simulink model "bldc_model_bst"  (R2014b)
settings: Solver=ode4  StartTime=0.0  StopTime=5  FixedStep=0.01  RelTol=1e-3
undefined symbols (not defined in the file or in its folder): spd_0
libraries: simulink x2
settings Model: Creator=root  LastModifiedBy=root

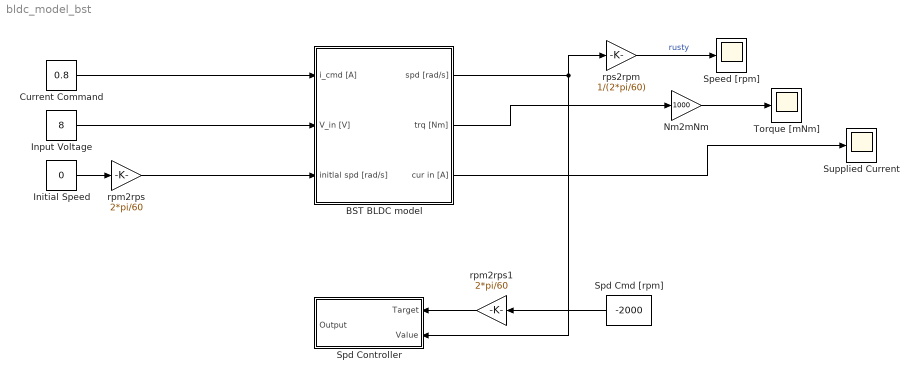
== system bldc_model_bst ==
  BST BLDC model : Subsystem  mask{Ke=1.026E-3/(2*pi/60), Km=1/96.154, R=2.3, frctn_c=[-3.77e-09, -1.42e-06, -6.76e-04], frctn_p=[-3.39e-09, -1.57e-06, -5.89e-04], frctn_n=[-9.44e-09, -4.31e-05, +3.57e-04], J=978.548e-6, i_max=0.9, V_in=8.0}
      mask prompts: Ke "Back-EMF Constant [V/(rad/s)]"; Km "Motor Torque Constant [Nm/A]"; R "Motor Resistance [Ohm]"; frctn_c "Friction Coefficients"; frctn_p "Friction Coefficients Pos"; frctn_n "Friction Coefficients Neg"; J "Moment of Inertia [kgm2]"; i_max "Maximum Current [A]"; V_in "Input Voltage [V]"
  "Current Command " : Constant  Value=0.8
  Initial Speed : Constant  Value=0
  Input Voltage : Constant  Value=8
  Nm2mNm : Gain  Gain=1000
  Spd Cmd [rpm] : Constant  Value=-2000
  Spd Controller : Subsystem  mask{kp=100E-3, ki=3.0e-05, kd=0.0, output_max=0.9}
      mask prompts: kp "Proportional Gain"; ki "Integrator Gain"; kd "Derivative Gain"; output_max "Maximum Output"
      mask DialogControl DescTextVar Prompt: This is a general PID controller with propotional gains, derivative gain and integral gain
  "Speed [rpm] " : Scope
      settings: ShowLegends=on  TimeRange=5  YMin=0  YMax=400
  Supplied Current : Scope
      settings: ShowLegends=on  TimeRange=10  YMin=0.344  YMax=0.351  SaveName=ScopeData2
  Torque [mNm] : Scope
      settings: ShowLegends=on  TimeRange=300  YMin=-20  YMax=20
  rpm2rps : Gain  Gain=2*pi/60
  rpm2rps1 : Gain  Gain=2*pi/60
  rps2rpm : Gain  Gain=1/(2*pi/60)
  wires:
  "Current Command "/1 -> BST BLDC model/1(i_cmd [A])
  BST BLDC model/1(spd [rad/s]) -> rps2rpm/1, Spd Controller/2(Value)
  rps2rpm/1 -> "Speed [rpm] "/1  "rusty"
  Input Voltage/1 -> BST BLDC model/2(V_in [V])
  Initial Speed/1 -> rpm2rps/1
  rpm2rps/1 -> BST BLDC model/3(initlal spd [rad/s])
  BST BLDC model/2(trq [Nm]) -> Nm2mNm/1
  Nm2mNm/1 -> Torque [mNm]/1
  BST BLDC model/3(cur in [A]) -> Supplied Current/1
  Spd Cmd [rpm]/1 -> rpm2rps1/1
  rpm2rps1/1 -> Spd Controller/1(Target)

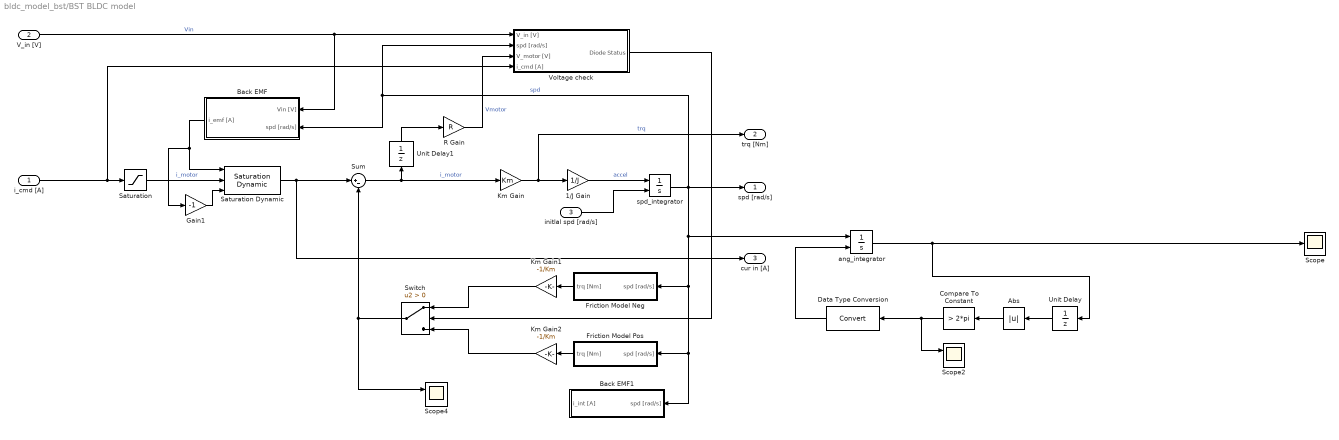
== system bldc_model_bst/BST BLDC model ==
  i_cmd [A] : Inport
  V_in [V] : Inport  Port=2
  initlal spd [rad/s] : Inport  Port=3
  1/J Gain : Gain  Gain=1/J
  Abs : Abs
  Back EMF : Subsystem
  Back EMF1 : Subsystem
  Compare To Constant : simulink/Logic and Bit Operations/Compare To Constant  relop=>  const=2*pi  OutDataTypeStr=uint8
  Data Type Conversion : DataTypeConversion
  Friction Model Neg : Subsystem  mask{frctn=frctn_n}
      mask prompts: frctn "Friction Coefficients"
  Friction Model Pos : Subsystem  mask{frctn=frctn_p}
      mask prompts: frctn "Friction Coefficients"
  Gain1 : Gain  Gain=-1
  Km Gain : Gain  Gain=Km
  Km Gain1 : Gain  Gain=-1/Km
  Km Gain2 : Gain  Gain=-1/Km
  R Gain : Gain  Gain=R
  Saturation : Saturate  UpperLimit=i_max  LowerLimit=-i_max
  Saturation Dynamic : simulink/Discontinuities/Saturation Dynamic  OutMin=[]  OutMax=[]  OutDataTypeStr=Inherit: Same as second input  OutDataType=fixdt(1, 16)  OutScaling=2^-10  DoSatur=off
  Scope : Scope
      settings: TimeRange=30  SaveName=ScopeData3
  Scope2 : Scope  NumInputPorts=2
      settings: TimeRange=30  YMin=-5~-5  YMax=5~5  SaveName=ScopeData7
  Scope4 : Scope  NumInputPorts=2
      settings: TimeRange=10  YMin=0~0  YMax=12~1.4  SaveName=ScopeData10
  Sum : Sum  Inputs=|+-
  Switch : Switch  Criteria=u2 > Threshold
  Unit Delay : UnitDelay  SampleTime=-1
  Unit Delay1 : UnitDelay  SampleTime=-1
  Voltage check : Subsystem
  ang_integrator : Integrator  ExternalReset=rising
  spd_integrator : Integrator  InitialConditionSource=external  InitialCondition=spd_0
  spd [rad/s] : Outport
  trq [Nm] : Outport  Port=2
  cur in [A] : Outport  Port=3
  wires:
  Km Gain/1 -> trq [Nm]/1, 1/J Gain/1  "trq"
  spd_integrator/1 -> ang_integrator/1, Back EMF1/1(spd [rad/s]), Friction Model Pos/1(spd [rad/s]), Friction Model Neg/1(spd [rad/s]), spd [rad/s]/1, Voltage check/2(spd [rad/s]), Back EMF/2(spd [rad/s])  "spd"
  Sum/1 -> Km Gain/1, Unit Delay1/1  "i_motor"
  i_cmd [A]/1 -> Voltage check/4(i_cmd [A]), Saturation/1
  Friction Model Neg/1(trq [Nm]) -> Km Gain1/1
  1/J Gain/1 -> spd_integrator/1  "accel"
  V_in [V]/1 -> Voltage check/1(V_in [V]), Back EMF/1(Vin [V])  "Vin"
  Saturation/1 -> Saturation Dynamic/2  "i_motor"
  Saturation Dynamic/1 -> cur in [A]/1, Sum/1
  Gain1/1 -> Saturation Dynamic/3
  Friction Model Pos/1(trq [Nm]) -> Km Gain2/1
  Unit Delay1/1 -> R Gain/1
  Back EMF/1(i_emf [A]) -> Saturation Dynamic/1, Gain1/1
  Km Gain2/1 -> Switch/3
  Km Gain1/1 -> Switch/1
  Voltage check/1(Diode Status) -> Switch/2
  R Gain/1 -> Voltage check/3(V_motor [V])  "Vmotor"
  initlal spd [rad/s]/1 -> spd_integrator/2
  Abs/1 -> Compare To Constant/1
  ang_integrator/1 -> Scope/1, Unit Delay/1
  Unit Delay/1 -> Abs/1
  Data Type Conversion/1 -> ang_integrator/2
  Compare To Constant/1 -> Scope2/1, Data Type Conversion/1
  Switch/1 -> Sum/2, Scope4/1

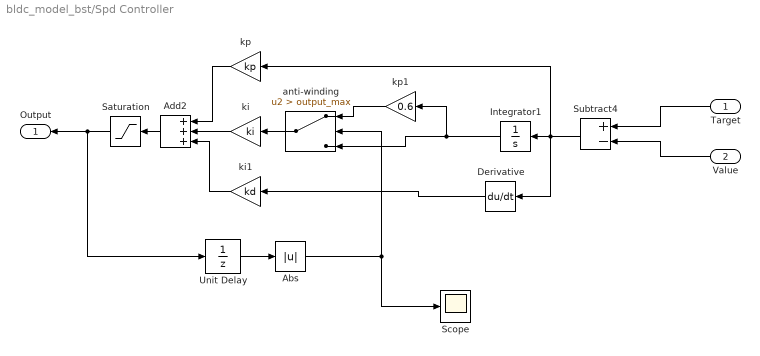
== system bldc_model_bst/Spd Controller ==
  Target : Inport
  Value : Inport  Port=2
  Abs : Abs
  Add2 : Sum  Inputs=+++
  Derivative : Derivative
  Integrator1 : Integrator
  Saturation : Saturate  UpperLimit=2  LowerLimit=-2
  Scope : Scope
      settings: SaveName=ScopeData6
  Subtract4 : Sum  Inputs=+-
  Unit Delay : UnitDelay  SampleTime=-1
  anti-winding : Switch  Criteria=u2 > Threshold  Threshold=output_max
  ki : Gain  Gain=ki
  ki1 : Gain  Gain=kd
  kp : Gain  Gain=kp
  kp1 : Gain  Gain=0.6
  Output : Outport
  wires:
  Target/1 -> Subtract4/1
  Value/1 -> Subtract4/2
  Integrator1/1 -> anti-winding/3, kp1/1
  kp/1 -> Add2/1
  ki/1 -> Add2/2
  Derivative/1 -> ki1/1
  ki1/1 -> Add2/3
  Subtract4/1 -> Integrator1/1, kp/1, Derivative/1
  anti-winding/1 -> ki/1
  kp1/1 -> anti-winding/1
  Abs/1 -> Scope/1, anti-winding/2
  Unit Delay/1 -> Abs/1
  Add2/1 -> Saturation/1
  Saturation/1 -> Output/1, Unit Delay/1

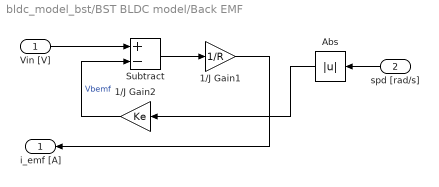
== system bldc_model_bst/BST BLDC model/Back EMF ==
  Vin [V] : Inport
  spd [rad/s] : Inport  Port=2
  1/J Gain1 : Gain  Gain=1/R
  1/J Gain2 : Gain  Gain=Ke
  Abs : Abs
  Subtract : Sum  Inputs=+-
  i_emf [A] : Outport
  wires:
  Vin [V]/1 -> Subtract/1
  1/J Gain1/1 -> i_emf [A]/1
  Subtract/1 -> 1/J Gain1/1
  spd [rad/s]/1 -> Abs/1
  1/J Gain2/1 -> Subtract/2  "Vbemf"
  Abs/1 -> 1/J Gain2/1

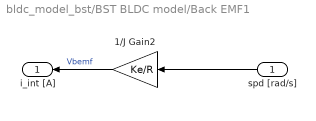
== system bldc_model_bst/BST BLDC model/Back EMF1 ==
  spd [rad/s] : Inport
  1/J Gain2 : Gain  Gain=Ke/R
  i_int [A] : Outport
  wires:
  1/J Gain2/1 -> i_int [A]/1  "Vbemf"
  spd [rad/s]/1 -> 1/J Gain2/1

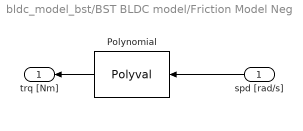
== system bldc_model_bst/BST BLDC model/Friction Model Neg ==
  spd [rad/s] : Inport
  Polynomial : Polyval  Coefs=frctn
  trq [Nm] : Outport
  wires:
  spd [rad/s]/1 -> Polynomial/1
  Polynomial/1 -> trq [Nm]/1

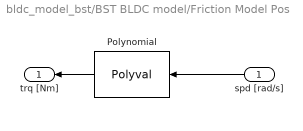
== system bldc_model_bst/BST BLDC model/Friction Model Pos ==
  spd [rad/s] : Inport
  Polynomial : Polyval  Coefs=frctn
  trq [Nm] : Outport
  wires:
  spd [rad/s]/1 -> Polynomial/1
  Polynomial/1 -> trq [Nm]/1

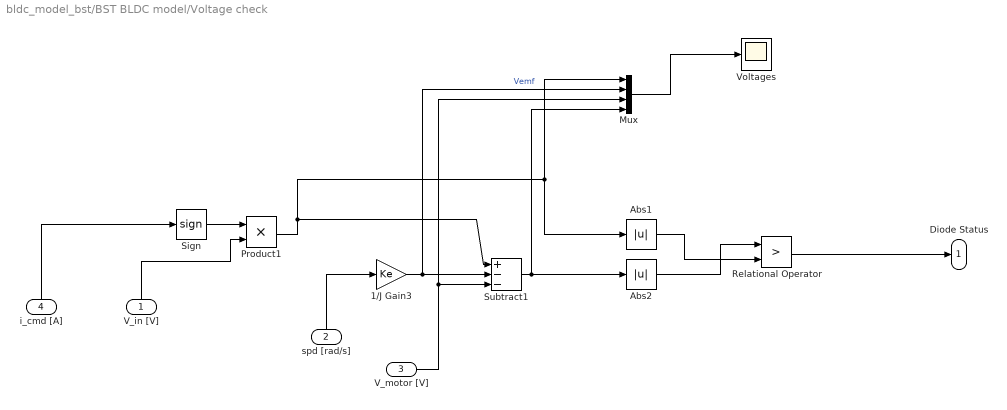
== system bldc_model_bst/BST BLDC model/Voltage check ==
  V_in [V] : Inport
  spd [rad/s] : Inport  Port=2
  V_motor [V] : Inport  Port=3
  i_cmd [A] : Inport  Port=4
  1/J Gain3 : Gain  Gain=Ke
  Abs1 : Abs
  Abs2 : Abs
  Mux : Mux
  Product1 : Product
  Relational Operator : RelationalOperator  Operator=>  OutDataTypeStr=boolean
  Sign : Signum
  Subtract1 : Sum  Inputs=+--
  Voltages : Scope
      settings: ShowLegends=on  TimeRange=30  YMin=-25  YMax=0  SaveName=ScopeData4  ScrollMode=on
  Diode Status : Outport
  wires:
  spd [rad/s]/1 -> 1/J Gain3/1
  Relational Operator/1 -> Diode Status/1
  1/J Gain3/1 -> Mux/2, Subtract1/2  "Vemf"
  Sign/1 -> Product1/1
  Subtract1/1 -> Mux/4, Abs2/1
  Abs2/1 -> Relational Operator/1
  V_motor [V]/1 -> Mux/3, Subtract1/3
  i_cmd [A]/1 -> Sign/1
  Abs1/1 -> Relational Operator/2
  V_in [V]/1 -> Product1/2
  Mux/1 -> Voltages/1
  Product1/1 -> Abs1/1, Mux/1, Subtract1/1
